simulink model "finalt3"  (R2021b)
settings: Solver=VariableStepAuto  StartTime=0.0  StopTime=tf  RelTol=1e-3
values from neighbouring files (symbols this model uses):
  alpha = 8    [Code_test3.m]
  beta = 8    [Code_test3.m]
  beta_d = 8    [Code_test3.m]
  c = 20 + (30-20).*rand(N,1)    [Code_test3.m]
  dwell_time = 15    [Code_test3.m]
  eta_dot_IC = [0, 0]'    [Code_test3.m]
  eta_IC = [105, -5]'    [Code_test3.m]
  f = 0.03    [Code_test3.m]
  Gamma = diag(Gamma)    [Code_test3.m]
  KCL = 0.01*Gamma    [Code_test3.m]
  m = 200 + (300-200).*rand(N,1)    [Code_test3.m]
  R = 100    [Code_test3.m]
  theta = [m, c]'    [Code_test3.m]
  theta_hat_IC = [init + (last+init)*rand(N,1), init + (last+init)*rand(N,1)]'    [Code_test3.m]
libraries: simulink x4
settings Model: Creator=kaush  LastModifiedBy=kaush

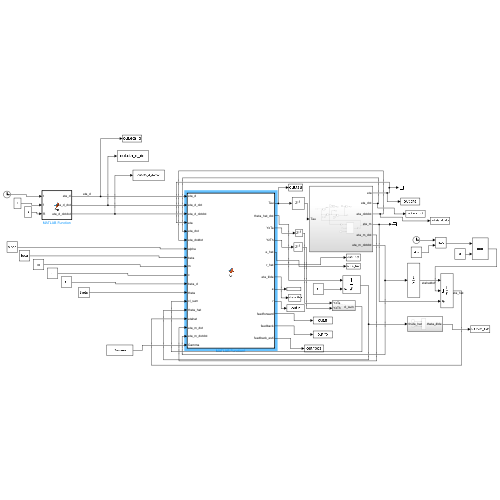
[thumbnail: Simulink's stored preview of the top-level diagram]
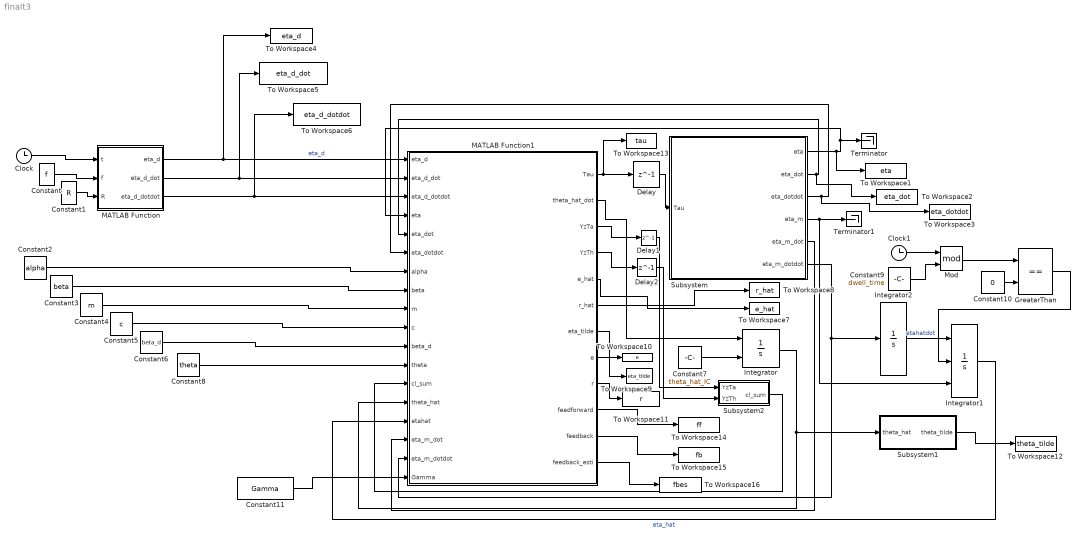
== system finalt3 ==
  Clock : Clock
  Clock1 : Clock
  Constant : Constant  Value=f
  Constant1 : Constant  Value=R
  Constant10 : Constant  Value=0
  Constant11 : Constant  Value=Gamma
  Constant2 : Constant  Value=alpha
  Constant3 : Constant  Value=beta
  Constant4 : Constant  Value=m
  Constant5 : Constant  Value=c
  Constant6 : Constant  Value=beta_d
  Constant7 : Constant  Value=theta_hat_IC
  Constant8 : Constant  Value=theta
  Constant9 : Constant  Value=dwell_time
  Delay : Delay  DelayLength=1
  Delay1 : Delay  DelayLength=1  InitialCondition=zeros(2,1)
  Delay2 : Delay  DelayLength=1  InitialCondition=zeros(2,1)
  GreaterThan : RelationalOperator  Operator===  OutDataTypeStr=boolean  RndMeth=Simplest
  Integrator : Integrator  InitialConditionSource=external
  Integrator1 : Integrator  ExternalReset=rising  InitialConditionSource=external
  Integrator2 : Integrator
  MATLAB Function : MATLAB Function  TreatAsAtomicUnit=on
  MATLAB Function1 : MATLAB Function  TreatAsAtomicUnit=on
  Mod : Math  Operator=mod  SaturateOnIntegerOverflow=on
  Subsystem : Subsystem
  Subsystem1 : Subsystem
  Subsystem2 : Subsystem
  Terminator : Terminator
  Terminator1 : Terminator
  To Workspace1 : ToWorkspace  VariableName=eta  SaveFormat=Timeseries  SampleTime=-1
  To Workspace10 : ToWorkspace  VariableName=e  SaveFormat=Timeseries  SampleTime=-1
  To Workspace11 : ToWorkspace  VariableName=r  SaveFormat=Timeseries  SampleTime=-1
  To Workspace12 : ToWorkspace  VariableName=theta_tilde  SaveFormat=Timeseries  SampleTime=-1
  To Workspace13 : ToWorkspace  VariableName=tau  SaveFormat=Timeseries  SampleTime=-1
  To Workspace14 : ToWorkspace  VariableName=ff  SaveFormat=Timeseries  SampleTime=-1
  To Workspace15 : ToWorkspace  VariableName=fb  SaveFormat=Timeseries  SampleTime=-1
  To Workspace16 : ToWorkspace  VariableName=fbes  SaveFormat=Timeseries  SampleTime=-1
  To Workspace2 : ToWorkspace  VariableName=eta_dot  SaveFormat=Timeseries  SampleTime=-1
  To Workspace3 : ToWorkspace  VariableName=eta_dotdot  SaveFormat=Timeseries  SampleTime=-1
  To Workspace4 : ToWorkspace  VariableName=eta_d  SaveFormat=Timeseries  SampleTime=-1
  To Workspace5 : ToWorkspace  VariableName=eta_d_dot  SaveFormat=Timeseries  SampleTime=-1
  To Workspace6 : ToWorkspace  VariableName=eta_d_dotdot  SaveFormat=Timeseries  SampleTime=-1
  To Workspace7 : ToWorkspace  VariableName=e_hat  SaveFormat=Timeseries  SampleTime=-1
  To Workspace8 : ToWorkspace  VariableName=r_hat  SaveFormat=Timeseries  SampleTime=-1
  To Workspace9 : ToWorkspace  VariableName=eta_tilde  SaveFormat=Timeseries  SampleTime=-1
  wires:
  Delay/1 -> Subsystem/1(Tau)
  MATLAB Function1/1(Tau) -> To Workspace13/1, Delay/1
  Constant5/1 -> MATLAB Function1/10(c)
  Constant2/1 -> MATLAB Function1/7(alpha)
  Constant3/1 -> MATLAB Function1/8(beta)
  Constant1/1 -> MATLAB Function/3(R)
  Constant/1 -> MATLAB Function/2(f)
  Clock/1 -> MATLAB Function/1(t)
  MATLAB Function/3(eta_d_dotdot) -> MATLAB Function1/3(eta_d_dotdot), To Workspace6/1
  MATLAB Function/2(eta_d_dot) -> MATLAB Function1/2(eta_d_dot), To Workspace5/1
  MATLAB Function/1(eta_d) -> MATLAB Function1/1(eta_d), To Workspace4/1  "eta_d"
  Constant6/1 -> MATLAB Function1/11(beta_d)
  Constant4/1 -> MATLAB Function1/9(m)
  MATLAB Function1/2(theta_hat_dot) -> Integrator/1
  Constant7/1 -> Integrator/2
  Integrator/1 -> Subsystem1/1(theta_hat), MATLAB Function1/14(theta_hat)
  MATLAB Function1/3(YzTa) -> Delay1/1
  MATLAB Function1/4(YzTh) -> Delay2/1
  Subsystem2/1(cl_sum) -> MATLAB Function1/13(cl_sum)
  Constant8/1 -> MATLAB Function1/12(theta)
  Subsystem/1(eta) -> To Workspace1/1, MATLAB Function1/4(eta), Terminator/1
  Delay1/1 -> Subsystem2/1(YzTa)
  Delay2/1 -> Subsystem2/2(YzTh)
  Subsystem/2(eta_dot) -> To Workspace2/1, MATLAB Function1/5(eta_dot)
  Subsystem/3(eta_dotdot) -> To Workspace3/1, MATLAB Function1/6(eta_dotdot)
  Subsystem/5(eta_m_dot) -> MATLAB Function1/16(eta_m_dot)
  Subsystem/6(eta_m_dotdot) -> Integrator2/1, MATLAB Function1/17(eta_m_dotdot)
  Subsystem/4(eta_m) -> Integrator1/3, Terminator1/1
  Integrator1/1 -> MATLAB Function1/15(etahat)  "eta_hat"
  Integrator2/1 -> Integrator1/1  "etahatdot"
  Clock1/1 -> Mod/1
  Constant9/1 -> Mod/2
  Mod/1 -> GreaterThan/1
  Constant10/1 -> GreaterThan/2
  GreaterThan/1 -> Integrator1/2
  Constant11/1 -> MATLAB Function1/18(Gamma)
  MATLAB Function1/5(e_hat) -> To Workspace7/1
  MATLAB Function1/6(r_hat) -> To Workspace8/1
  MATLAB Function1/7(eta_tilde) -> To Workspace9/1
  MATLAB Function1/9(r) -> To Workspace11/1
  MATLAB Function1/8(e) -> To Workspace10/1
  Subsystem1/1(theta_tilde) -> To Workspace12/1
  MATLAB Function1/10(feedforward) -> To Workspace14/1
  MATLAB Function1/12(feedback_esti) -> To Workspace16/1
  MATLAB Function1/11(feedback) -> To Workspace15/1

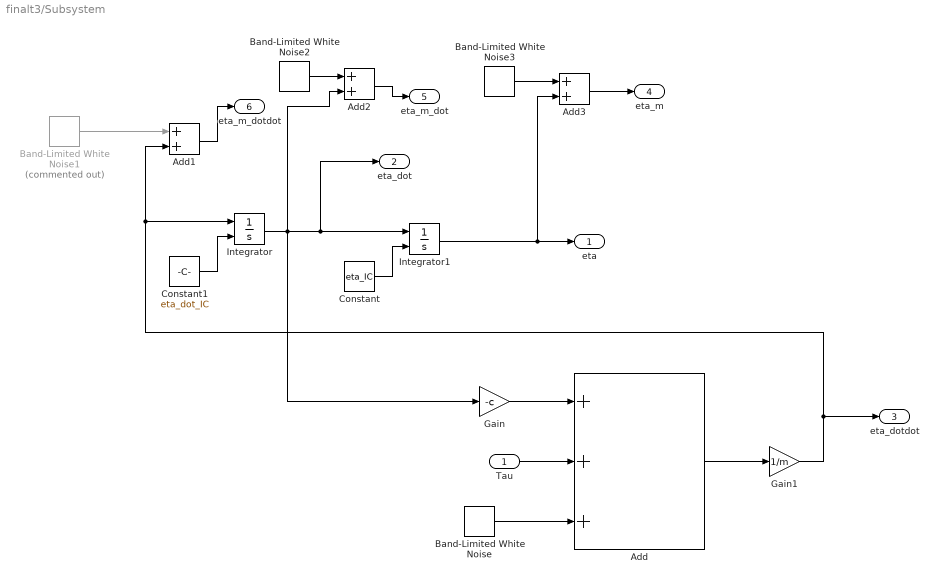
== system finalt3/Subsystem ==
  Tau : Inport
  Add : Sum  Inputs=+++
  Add1 : Sum
  Add2 : Sum
  Add3 : Sum
  Band-Limited White Noise : simulink/Sources/Band-Limited White Noise  Cov=[0.00001]  Ts=0.1  seed=[23341]
  Band-Limited White Noise1 : simulink/Sources/Band-Limited White Noise  Commented=on  Cov=[0.00001]  Ts=0.1  seed=[23341]
  Band-Limited White Noise2 : simulink/Sources/Band-Limited White Noise  Cov=[0.00001]  Ts=0.1  seed=[23341]
  Band-Limited White Noise3 : simulink/Sources/Band-Limited White Noise  Cov=[0.00001]  Ts=0.1  seed=[23341]
  Constant : Constant  Value=eta_IC
  Constant1 : Constant  Value=eta_dot_IC
  Gain : Gain  Gain=-c
  Gain1 : Gain  Gain=1/m
  Integrator : Integrator  InitialConditionSource=external
  Integrator1 : Integrator  InitialConditionSource=external
  eta : Outport
  eta_dot : Outport  Port=2
  eta_dotdot : Outport  Port=3
  eta_m : Outport  Port=4
  eta_m_dot : Outport  Port=5
  eta_m_dotdot : Outport  Port=6
  wires:
  Integrator/1 -> Add2/2, Gain/1, eta_dot/1, Integrator1/1
  Constant/1 -> Integrator1/2
  Constant1/1 -> Integrator/2
  Integrator1/1 -> Add3/2, eta/1
  Gain/1 -> Add/1
  Tau/1 -> Add/2
  Band-Limited White Noise/1 -> Add/3
  Add/1 -> Gain1/1
  Band-Limited White Noise1/1 -> Add1/1
  Gain1/1 -> eta_dotdot/1, Integrator/1, Add1/2
  Add1/1 -> eta_m_dotdot/1
  Band-Limited White Noise2/1 -> Add2/1
  Add2/1 -> eta_m_dot/1
  Band-Limited White Noise3/1 -> Add3/1
  Add3/1 -> eta_m/1

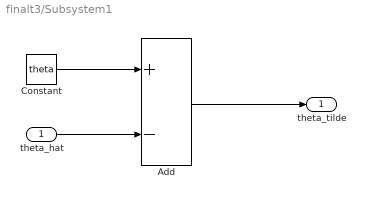
== system finalt3/Subsystem1 ==
  theta_hat : Inport
  Add : Sum  Inputs=+-
  Constant : Constant  Value=theta
  theta_tilde : Outport
  wires:
  Constant/1 -> Add/1
  theta_hat/1 -> Add/2
  Add/1 -> theta_tilde/1

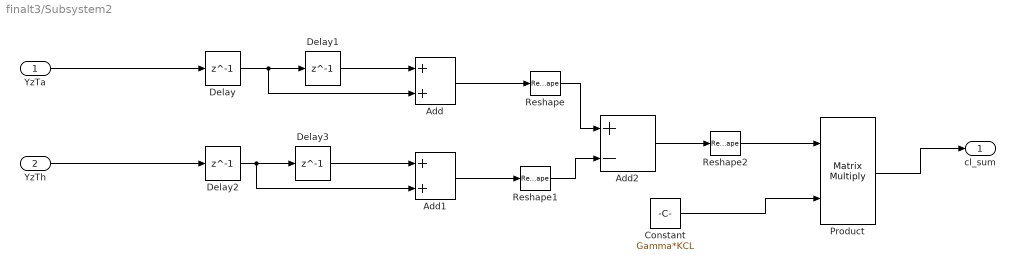
== system finalt3/Subsystem2 ==
  YzTa : Inport
  YzTh : Inport  Port=2
  Add : Sum
  Add1 : Sum
  Add2 : Sum  Inputs=+-
  Constant : Constant  Value=Gamma*KCL
  Delay{,1..3} (4 alike) : Delay  DelayLength=1
  Product : Product  Multiplication=Matrix(*)
  Reshape : Reshape  OutputDimensionality=Row vector (2-D)
  Reshape1 : Reshape  OutputDimensionality=Row vector (2-D)
  Reshape2 : Reshape  OutputDimensionality=Row vector (2-D)
  cl_sum : Outport
  wires:
  Delay1/1 -> Add/1
  Delay/1 -> Add/2, Delay1/1
  Delay3/1 -> Add1/1
  Delay2/1 -> Add1/2, Delay3/1
  Add/1 -> Reshape/1
  Add1/1 -> Reshape1/1
  Reshape/1 -> Add2/1
  Reshape1/1 -> Add2/2
  Add2/1 -> Reshape2/1
  Constant/1 -> Product/2
  Product/1 -> cl_sum/1
  YzTa/1 -> Delay/1
  YzTh/1 -> Delay2/1
  Reshape2/1 -> Product/1

== matlab function finalt3/MATLAB Function1 ==
  data: eta_d input; Tau output; eta_d_dot input; eta_d_dotdot input; eta input; eta_dot input; eta_dotdot input; alpha input; beta input; m input; c input; beta_d input; theta input; cl_sum input; theta_hat input; theta_hat_dot output; YzTa output; YzTh output; etahat input; eta_m_dot input; eta_m_dotdot input; Gamma input; e_hat output; r_hat output; eta_tilde output; e output; r output; feedforward output; feedback output; feedback_esti output
function [Tau, theta_hat_dot, YzTa, YzTh, e_hat, r_hat, eta_tilde, e, r, feedforward, feedback, feedback_esti] = fcn(eta_d, eta_d_dot, eta_d_dotdot, eta, eta_dot, eta_dotdot, alpha, beta, m, c, beta_d, theta, cl_sum, theta_hat, etahat, eta_m_dot, eta_m_dotdot, Gamma)



% e_hat_dot = [1e-2, 2e-1]';
% r_hat = [1e-1, 2e-3]';
% Y = [[1e-1, 2e-3]', [1e-2, 2e-1]'];
% Tau = [1e-1, 2e-1]';
%etahat = eta;
e = eta_d - eta;
e_dot = eta_d_dot - eta_dot;
r = e_dot + alpha*e;
e_hat = eta_d - etahat;
e_hat_dot = eta_d_dot - eta_dot;
% r = e_dot + alpha*e_hat;
eta_tilde = eta - etahat;
e_hat_dot = eta_d_dot - eta_m_dot;
r_hat = e_hat_dot + alpha*e_hat;
Y = [(alpha*e_hat_dot + eta_d_dotdot), (eta_dot)];
Tau = Y*theta_hat + e_hat+ beta*r_hat + beta_d*sign(r_hat);
Y_z = [(eta_dotdot), (eta_dot)];
YzTa = Y_z'*Tau;
YzTh = Y_z'*Y_z*theta_hat;
theta_hat_dot = Gamma*Y'*r_hat + cl_sum';
feedforward = Y*theta_hat;
feedback = e + beta*r;
%feedforward = Y*theta_hat;
feedback_esti = e_hat + beta*r_hat;

== matlab function finalt3/MATLAB Function ==
  data: t input; eta_d output; f input; R input; eta_d_dot output; eta_d_dotdot output
function [eta_d, eta_d_dot, eta_d_dotdot]= fcn(t,f,R)
eta_d = R*[cos(2*pi*f*t); sin(2*pi*f*t)];
eta_d_dot = 2*pi*f*R*[-sin(2*pi*f*t); cos(2*pi*f*t)];
eta_d_dotdot = (2*pi*f)*(2*pi*f)*R*[-cos(2*pi*f*t); -sin(2*pi*f*t)];
